simulink model "bloco_question1_v1"  (Simulink 7.1)
settings: Solver=ode45  StartTime=0.0  StopTime=10.0  RelTol=1e-3
settings Model: Creator=ALUNO  LastModifiedBy=ALUNO

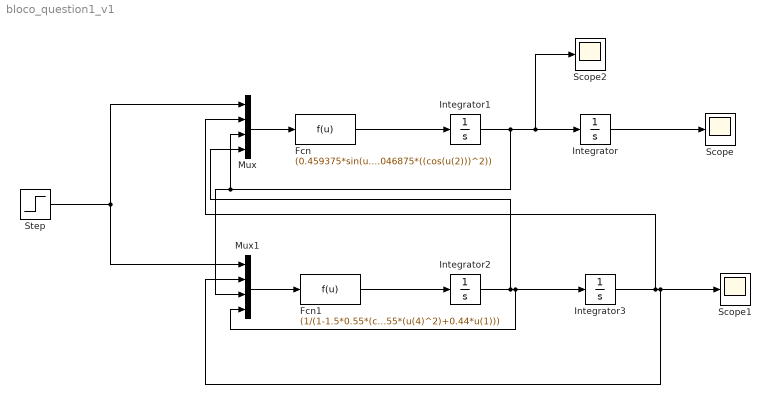
== system bloco_question1_v1 ==
  Fcn : Fcn  Expr=(0.459375*sin(u(2))*cos(u(2)) -0.125*u(3) + 0.0325*(u(4)^2)*sin(u(2)) + 0.25*u(1))/(0.5625 - 0.046875*((cos(u(2)))^2))
  Fcn1 : Fcn  Expr=(1/(1-1.5*0.55*(cos(u(2))^2)))*(-14.71*sin(u(2))-1.5*cos(u(2))*(-0.22*u(3)+0.055*(u(4)^2)+0.44*u(1)))
  Integrator : Integrator
  Integrator1 : Integrator
  Integrator2 : Integrator
  Integrator3 : Integrator  InitialCondition=(pi/6)
  Mux : Mux
  Mux1 : Mux
  Scope : Scope
  Scope1 : Scope
  Scope2 : Scope
      settings: SaveName=ScopeData2
  Step : Step  After=0  SampleTime=0
  wires:
  Mux/1 -> Fcn/1
  Mux1/1 -> Fcn1/1
  Fcn/1 -> Integrator1/1
  Integrator1/1 -> Mux/3, Mux1/3, Integrator/1, Scope2/1
  Fcn1/1 -> Integrator2/1
  Integrator2/1 -> Mux/4, Integrator3/1, Mux1/4
  Integrator/1 -> Scope/1
  Integrator3/1 -> Mux/2, Scope1/1, Mux1/2
  Step/1 -> Mux/1, Mux1/1
